simulink model "Estabilizacao_Moto"  (R2018a)
settings: Solver=ode45  StartTime=0.0  StopTime=20  MaxStep=0.001  RelTol=1e-3  EnableMultiTasking=on
values from neighbouring files (symbols this model uses):
  C = [1 1 1; 1 1 1]    [Filtro_Kalman.m]    (also in Filtro_Kalman_Estendido.m)
  Ts = 0.001    [Filtro_Kalman_Estendido.m]
undefined symbols (not defined in the file or in its folder): K, P0, sigbuilder_block, x0, x0obs
settings Model: Creator=hector  LastModifiedBy=antoniataveira
settings DataIOCC: LimitDataPoints=on  SaveFormat=Array
settings OptimizationCC: LifeSpan=inf
settings DebuggingCC: SolverPrmCheckMsg=warning  SFUnexpectedBacktrackingDiag=warning  SFNoUnconditionalDefaultTransitionDiag=warning  SFExecutionAtInitializationDiag=none
settings HardwareCC: ProdBitPerPointer=32  ProdBitPerSizeT=32  ProdBitPerPtrDiffT=32  ProdLargestAtomicFloat=None  ProdIntDivRoundTo=Undefined  ProdEndianess=Unspecified  ProdWordSize=32  ProdHWDeviceType=32-bit Generic
settings ModelReferenceCC: PropagateSignalLabelsOutOfModel=off
settings CodeAppCC: StateflowObjectComments=on
settings GRTTargetCC: TargetLangStandard=C89/C90 (ANSI)  GeneratePreprocessorConditionals=Disable all
settings ConfigComp: CovMetricSettings=dw  CovHtmlReporting=on  CovSaveCumulativeToWorkspaceVar=on  CovSaveSingleToWorkspaceVar=on  CovExternalEMLEnable=off  CovSFcnEnable=off

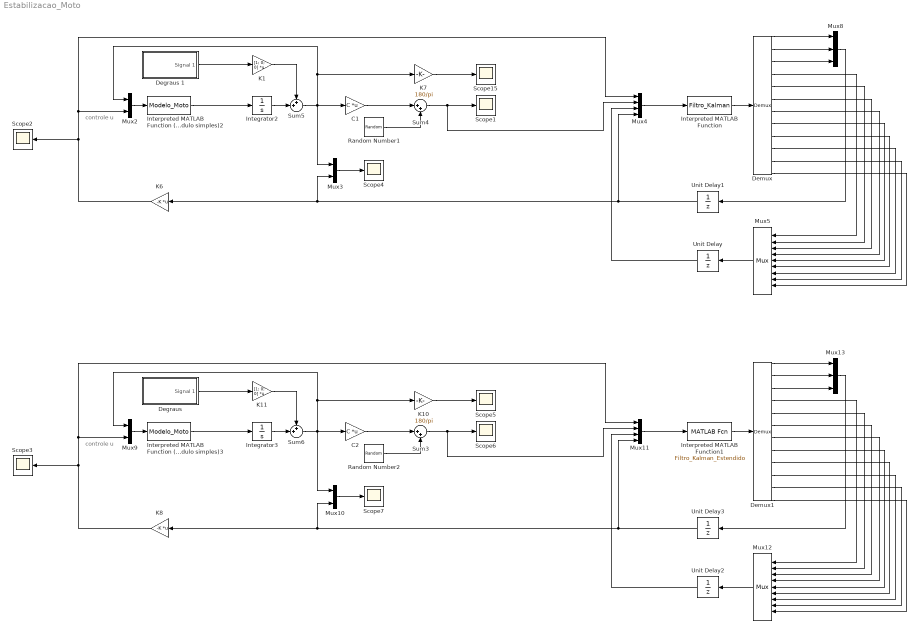
== system Estabilizacao_Moto ==
  note: controle u
  note: controle u
  C1 : Gain  Gain=C  Multiplication=Matrix(K*u)
  C2 : Gain  Gain=C  Multiplication=Matrix(K*u)
  "Degraus " : Subsystem  Tag=STV Subsys  LoadFcn=sigbuilder_block('load');  StartFcn=sigbuilder_block('start');  StopFcn=sigbuilder_block('stop');  ClipboardFcn=sigbuilder_block('clipboard');  mask(Sigbuilder block){tuvar=[0:10]}
      mask help: Simulink:masks:SigbuilderBlock_MD
      mask init:
      | if ~strcmp(get_param(bdroot(gcbh),'SimulationStatus'),'stopped') tuvar = sigbuilder_block('maskInit'); end
      settings: CopyFcn=sigbuilder_block('copy');  DeleteFcn=sigbuilder_block('delete');  ModelCloseFcn=sigbuilder_block('modelClose');  PreSaveFcn=sigbuilder_block('preSave');  PauseFcn=sigbuilder_block('pause');  ContinueFcn=sigbuilder_block('continue');  NameChangeFcn=sigbuilder_block('namechange');  OpenFcn=sigbuilder_block('open',[237 75 1437 799 ]);  CloseFcn=sigbuilder_block('close');
      mask Display: plot(0, 0, 100, 100,[2, 2, 32, 32, 2], [68, 8, 8, 68, 68],[32, 2], [38, 38], [32, 19, 2],[53, 60, 44], [32, 17, 17, 2],[16, 16, 31, 31]);txt = getActiveGroup(gcbh);text(2, 100, txt,'verticalAlignment', 'top');
  Degraus 1 : Subsystem  Tag=STV Subsys  LoadFcn=sigbuilder_block('load');  StartFcn=sigbuilder_block('start');  StopFcn=sigbuilder_block('stop');  ClipboardFcn=sigbuilder_block('clipboard');  mask(Sigbuilder block){tuvar=[0:10]}
      mask help: Simulink:masks:SigbuilderBlock_MD
      mask init:
      | if ~strcmp(get_param(bdroot(gcbh),'SimulationStatus'),'stopped') tuvar = sigbuilder_block('maskInit'); end
      settings: CopyFcn=sigbuilder_block('copy');  DeleteFcn=sigbuilder_block('delete');  ModelCloseFcn=sigbuilder_block('modelClose');  PreSaveFcn=sigbuilder_block('preSave');  PauseFcn=sigbuilder_block('pause');  ContinueFcn=sigbuilder_block('continue');  NameChangeFcn=sigbuilder_block('namechange');  OpenFcn=sigbuilder_block('open',[0 3.9937 1594.49 798.74 ]);  CloseFcn=sigbuilder_block('close');
      mask Display: plot(0, 0, 100, 100,[2, 2, 32, 32, 2], [68, 8, 8, 68, 68],[32, 2], [38, 38], [32, 19, 2],[53, 60, 44], [32, 17, 17, 2],[16, 16, 31, 31]);txt = getActiveGroup(gcbh);text(2, 100, txt,'verticalAlignment', 'top');
  Demux : Demux  Outputs=12
  Demux1 : Demux  Outputs=12
  Integrator2 : Integrator  InitialCondition=x0
  Integrator3 : Integrator  InitialCondition=x0
  Interpreted MATLAB Function : MATLABFcn  MATLABFcn=Filtro_Kalman  OutputDimensions=12  SampleTime=Ts
  Interpreted MATLAB Function (pendulo simples)2 : MATLABFcn  MATLABFcn=Modelo_Moto  OutputDimensions=3
  Interpreted MATLAB Function (pendulo simples)3 : MATLABFcn  MATLABFcn=Modelo_Moto  OutputDimensions=3
  Interpreted MATLAB Function1 : MATLABFcn  MATLABFcn=Filtro_Kalman_Estendido  OutputDimensions=12  SampleTime=Ts
  K1 : Gain  Gain=[1; 0; 0]  Multiplication=Matrix(K*u)
  K10 : Gain  Gain=180/pi
  K11 : Gain  Gain=[1; 0; 0]  Multiplication=Matrix(K*u)
  K6 : Gain  Gain=-K  Multiplication=Matrix(K*u)
  K7 : Gain  Gain=180/pi
  K8 : Gain  Gain=-K  Multiplication=Matrix(K*u)
  Mux{2..3,9..10} (4 alike) : Mux  Inputs=2
  Mux11 : Mux
  Mux12 : Mux  Inputs=9
  Mux13 : Mux  Inputs=3
  Mux4 : Mux
  Mux5 : Mux  Inputs=9
  Mux8 : Mux  Inputs=3
  Random Number1 : RandomNumber  Variance=0.00001  SampleTime=Ts
  Random Number2 : RandomNumber  Variance=0.00001  SampleTime=Ts
  Scope{1..7,15} (8 alike) : Scope
  Sum3 : Sum  Inputs=|++
  Sum4 : Sum  Inputs=|++
  Sum5 : Sum  Inputs=++|
  Sum6 : Sum  Inputs=++|
  Unit Delay : UnitDelay  InitialCondition=P0  SampleTime=Ts
  Unit Delay1 : UnitDelay  InitialCondition=x0obs  SampleTime=Ts
  Unit Delay2 : UnitDelay  InitialCondition=P0  SampleTime=Ts
  Unit Delay3 : UnitDelay  InitialCondition=x0obs  SampleTime=Ts
  wires:
  Mux2/1 -> Interpreted MATLAB Function (pendulo simples)2/1
  Interpreted MATLAB Function (pendulo simples)2/1 -> Integrator2/1
  K6/1 -> Scope2/1, Mux2/2, Mux4/1
  K7/1 -> Scope15/1
  C1/1 -> Sum4/1
  Sum4/1 -> Scope1/1, Mux4/2
  Random Number1/1 -> Sum4/2
  Sum5/1 -> Mux3/1, K7/1, Mux2/1, C1/1
  Integrator2/1 -> Sum5/2
  Mux4/1 -> Interpreted MATLAB Function/1
  Unit Delay/1 -> Mux4/3
  Unit Delay1/1 -> Mux3/2, K6/1, Mux4/4
  Interpreted MATLAB Function/1 -> Demux/1
  Mux5/1 -> Unit Delay/1
  Demux/1 -> Mux8/1
  Demux/2 -> Mux8/2
  Mux8/1 -> Unit Delay1/1
  Demux/4 -> Mux5/1
  Demux/5 -> Mux5/2
  Demux/6 -> Mux5/3
  Demux/7 -> Mux5/4
  Demux/8 -> Mux5/5
  Demux/9 -> Mux5/6
  Demux/10 -> Mux5/7
  Demux/11 -> Mux5/8
  Demux/12 -> Mux5/9
  Demux/3 -> Mux8/3
  Mux3/1 -> Scope4/1
  Mux9/1 -> Interpreted MATLAB Function (pendulo simples)3/1
  Interpreted MATLAB Function (pendulo simples)3/1 -> Integrator3/1
  K8/1 -> Scope3/1, Mux9/2, Mux11/1
  K10/1 -> Scope5/1
  C2/1 -> Sum3/1
  Sum3/1 -> Scope6/1, Mux11/2
  Random Number2/1 -> Sum3/2
  Sum6/1 -> Mux10/1, K10/1, Mux9/1, C2/1
  Integrator3/1 -> Sum6/2
  Mux11/1 -> Interpreted MATLAB Function1/1
  Unit Delay2/1 -> Mux11/3
  Unit Delay3/1 -> Mux10/2, K8/1, Mux11/4
  Interpreted MATLAB Function1/1 -> Demux1/1
  Mux12/1 -> Unit Delay2/1
  Demux1/1 -> Mux13/1
  Demux1/2 -> Mux13/2
  Mux13/1 -> Unit Delay3/1
  Demux1/4 -> Mux12/1
  Demux1/5 -> Mux12/2
  Demux1/6 -> Mux12/3
  Demux1/7 -> Mux12/4
  Demux1/8 -> Mux12/5
  Demux1/9 -> Mux12/6
  Demux1/10 -> Mux12/7
  Demux1/11 -> Mux12/8
  Demux1/12 -> Mux12/9
  Demux1/3 -> Mux13/3
  Mux10/1 -> Scope7/1
  "Degraus "/1(Signal 1) -> K11/1
  K11/1 -> Sum6/1
  Degraus 1/1(Signal 1) -> K1/1
  K1/1 -> Sum5/1

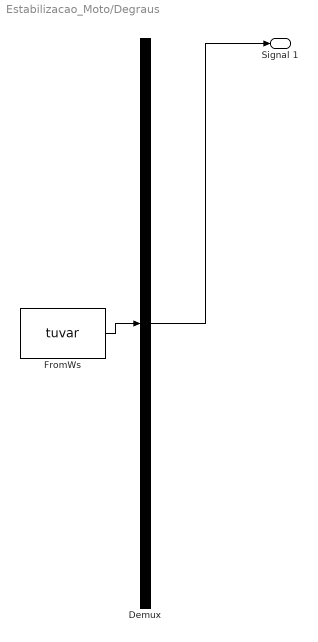
== system Estabilizacao_Moto/Degraus  ==
  Demux : Demux  Tag=STV Demux  Outputs=1
  FromWs : FromWorkspace  Tag=STV FromWs  VariableName=tuvar  SampleTime=0
      SigBuilderData=|
      | common.afterFinalStr = 'Extrapolate'
      | common.sampleTime = 0
      | dataSet.timeRange = [0 20]
      | dataSet.name = 'Group 1'
      | sbobj.Groups.Name = 'Group 1'
      | sbobj.Groups.Signals.Name = 'Signal 1'
      | sbobj.Groups.Signals.XData = [0 1.8 4 4 10 10 16 16 20]
      | sbobj.Groups.Signals.YData = [0 0 0 0.695 0.695 -0.3 -0.3 0.1 0.1]
      | sbobj.Groups.TimeRange = [0 20]
  Signal 1 : Outport  Tag=STV Outport
  wires:
  Demux/1 -> Signal 1/1
  FromWs/1 -> Demux/1

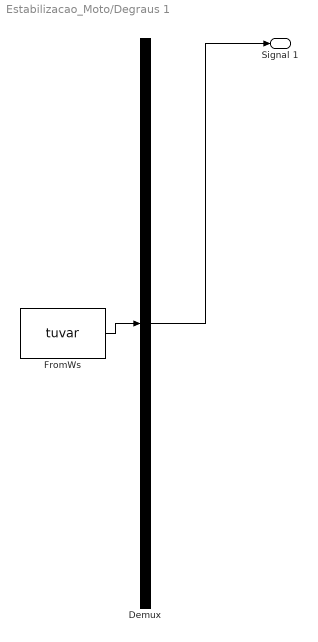
== system Estabilizacao_Moto/Degraus 1 ==
  Demux : Demux  Tag=STV Demux  Outputs=1
  FromWs : FromWorkspace  Tag=STV FromWs  VariableName=tuvar  SampleTime=0
      SigBuilderData=|
      | common.afterFinalStr = 'Extrapolate'
      | common.sampleTime = 0
      | dataSet.timeRange = [0 20]
      | dataSet.name = 'Group 1'
      | sbobj.Groups.Name = 'Group 1'
      | sbobj.Groups.Signals.Name = 'Signal 1'
      | sbobj.Groups.Signals.XData = [0 1.8 4 4 10 10 16 16 20]
      | sbobj.Groups.Signals.YData = [0 0 0 0.695 0.695 -0.3 -0.3 0.1 0.1]
      | sbobj.Groups.TimeRange = [0 20]
  Signal 1 : Outport  Tag=STV Outport
  wires:
  Demux/1 -> Signal 1/1
  FromWs/1 -> Demux/1
